simulink subsystem "DiagnosticManagement"  (R2019b)
settings: Solver=VariableStepAuto  StartTime=0.0  StopTime=10.0  RelTol=1e-3
settings Model: Creator=Nick  LastModifiedBy=Nick

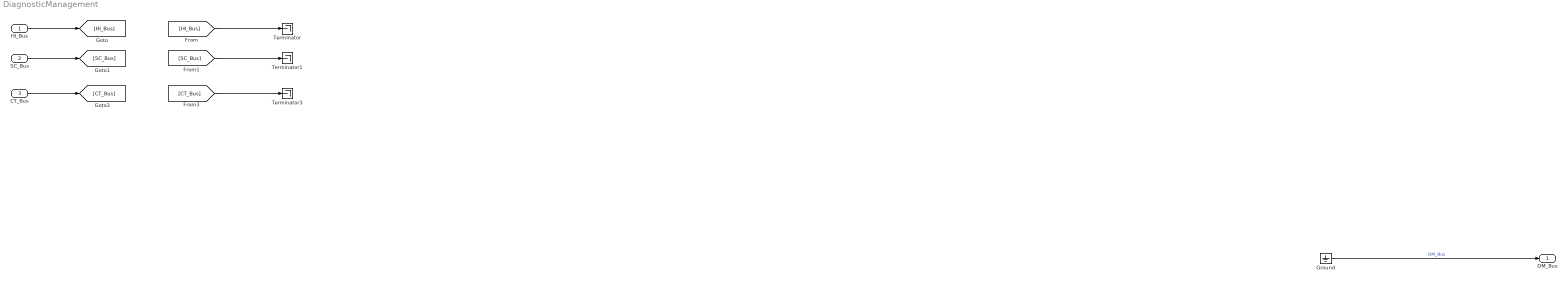
== system DiagnosticManagement ==
  HI_Bus : Inport
  SC_Bus : Inport  Port=2
  CT_Bus : Inport  Port=3
  Ground : Ground
  Terminator : Terminator
  Terminator1 : Terminator
  Terminator3 : Terminator
  DM_Bus : Outport
  wires:
  [HI_Bus] -> Terminator/1
  [SC_Bus] -> Terminator1/1
  HI_Bus/1 -> [HI_Bus]
  SC_Bus/1 -> [SC_Bus]
  Ground/1 -> DM_Bus/1  "DM_Bus"
  [CT_Bus] -> Terminator3/1
  CT_Bus/1 -> [CT_Bus]
